simulink model "exercise_07_simscape"  (R2022b)
settings: Solver=VariableStepAuto  StartTime=0.0  StopTime=10*2*pi/w  MaxStep=(2*pi/w)*1e-4  MinStep=(2*pi/w)*1e-12  RelTol=1e-3  AbsTol=1e-3
model workspace (MAT data in the model file):
  R = 1
  X1 = 1
  X2 = 2
  XC = -1
  XM = 1
  gamma1 = 1
  gamma2 = 1
  w = 6.28318530718
libraries: fl_lib x13, nesl_utility x5
settings Model: Creator=stefa  LastModifiedBy=stefa
settings SolverCC: AutoScaleAbsTol=off  AlgebraicLoopSolver=TrustRegion  MaxZcPerStep=1
settings OptimizationCC: ReuseModelBlockBuffer=on
settings DebuggingCC: UnconnectedInputMsg=warning  UnconnectedOutputMsg=warning  UnconnectedLineMsg=warning  SymbolicDimsDataTypeCodeGenerationDiagnostic=none
settings ModelReferenceCC: EnableRefExpFcnMdlSchedulingChecks=on
settings SFSimCC: CustomCodeUndefinedFunction=UseInterfaceOnly
settings RTWCC: DLArmComputeVersion=19.05
settings SimscapeCC: SimscapeLogType=all  SimscapeLogSimulationStatistics=on  SimscapeLogDataHistory=10000

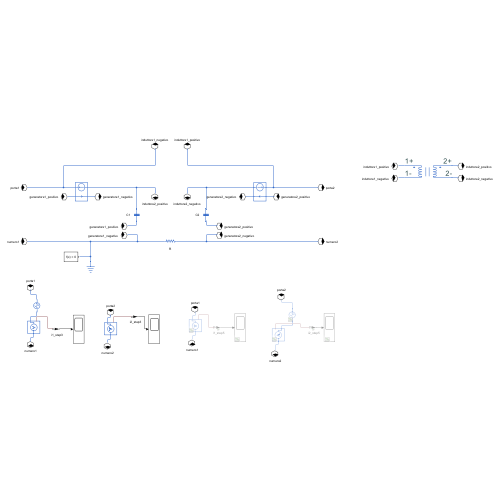
[thumbnail: Simulink's stored preview of the top-level diagram]
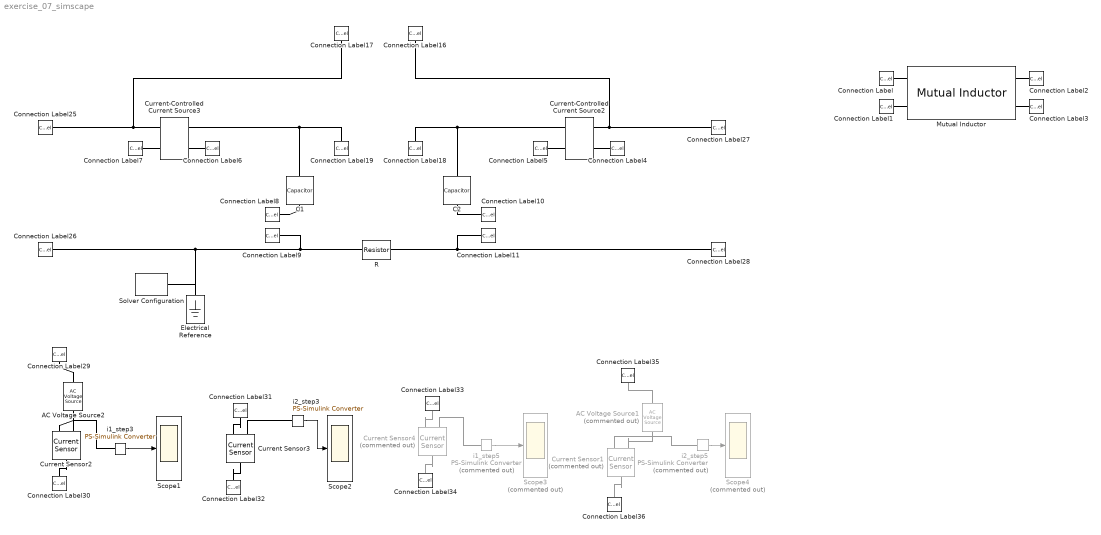
== system exercise_07_simscape ==
  AC Voltage Source1 : fl_lib/Electrical/Electrical Sources/AC Voltage Source  Commented=on  amp=1 V  shift=90 deg  frequency=w/(2*pi) Hz  omega=0 rad/s
  AC Voltage Source2 : fl_lib/Electrical/Electrical Sources/AC Voltage Source  amp=1 V  shift=90 deg  frequency=w/(2*pi) Hz  omega=0 rad/s
  C1 : fl_lib/Electrical/Electrical Elements/Capacitor  c=-1/w*XC F  r=0 Ohm  g=0 1/Ohm  i_specify=off  i_priority=None  i=0 A  i_nominal_specify=off  i_nominal_unit=A  i_nominal_value=1  v_specify=off  v_priority=None  v=0 V  v_nominal_specify=off  v_nominal_unit=V  v_nominal_value=1  vc_specify=off  vc_priority=High  vc=0 V  vc_nominal_specify=off  vc_nominal_unit=V  vc_nominal_value=1
  C2 : fl_lib/Electrical/Electrical Elements/Capacitor  c=-1/w*XC F  r=0 Ohm  g=0 1/Ohm  i_specify=off  i_priority=None  i=0 A  i_nominal_specify=off  i_nominal_unit=A  i_nominal_value=1  v_specify=off  v_priority=None  v=0 V  v_nominal_specify=off  v_nominal_unit=V  v_nominal_value=1  vc_specify=off  vc_priority=High  vc=0 V  vc_nominal_specify=off  vc_nominal_unit=V  vc_nominal_value=1
  Connection Label : ConnectionLabel  Label=induttore1_positivo
  Connection Label1 : ConnectionLabel  Label=induttore1_negativo
  Connection Label10 : ConnectionLabel  Label=generatore2_positivo
  Connection Label11 : ConnectionLabel  Label=generatore2_negativo
  Connection Label16 : ConnectionLabel  Label=induttore1_positivo
  Connection Label17 : ConnectionLabel  Label=induttore1_negativo
  Connection Label18 : ConnectionLabel  Label=induttore2_negativo
  Connection Label19 : ConnectionLabel  Label=induttore2_positivo
  Connection Label2 : ConnectionLabel  Label=induttore2_positivo
  Connection Label25 : ConnectionLabel  Label=porta1
  Connection Label26 : ConnectionLabel  Label=numero1
  Connection Label27 : ConnectionLabel  Label=porta2
  Connection Label28 : ConnectionLabel  Label=numero2
  Connection Label29 : ConnectionLabel  Label=porta1
  Connection Label3 : ConnectionLabel  Label=induttore2_negativo
  Connection Label30 : ConnectionLabel  Label=numero1
  Connection Label31 : ConnectionLabel  Label=porta2
  Connection Label32 : ConnectionLabel  Label=numero2
  Connection Label33 : ConnectionLabel  Label=porta1
  Connection Label34 : ConnectionLabel  Label=numero1
  Connection Label35 : ConnectionLabel  Label=porta2
  Connection Label36 : ConnectionLabel  Label=numero2
  Connection Label4 : ConnectionLabel  Label=generatore2_positivo
  Connection Label5 : ConnectionLabel  Label=generatore2_negativo
  Connection Label6 : ConnectionLabel  Label=generatore1_negativo
  Connection Label7 : ConnectionLabel  Label=generatore1_positivo
  Connection Label8 : ConnectionLabel  Label=generatore1_positivo
  Connection Label9 : ConnectionLabel  Label=generatore1_negativo
  Current Sensor1 : fl_lib/Electrical/Electrical Sensors/Current Sensor  Commented=on
  Current Sensor2 : fl_lib/Electrical/Electrical Sensors/Current Sensor
  Current Sensor3 : fl_lib/Electrical/Electrical Sensors/Current Sensor
  Current Sensor4 : fl_lib/Electrical/Electrical Sensors/Current Sensor  Commented=on
  Current-Controlled Current Source2 : fl_lib/Electrical/Electrical Sources/Current-Controlled Current Source  K=gamma2  i1_specify=off  i1_priority=None  i1=0 A  i1_nominal_specify=off  i1_nominal_unit=A  i1_nominal_value=1  i2_specify=off  i2_priority=None  i2=0 A  i2_nominal_specify=off  i2_nominal_unit=A  i2_nominal_value=1
      settings: InternalSimscapePortConfiguration="{\"Bottom\":[],\"Left\":[{\"id\":\"p1\",\"label\":\"+\",\"type\":\"foundation.electrical.electrical\"},{\"id\":\"head\",\"label\":\"\",\"type\":\"foundation.electrical.electrical\"}],\"Right\":[{\"id\":\"n1\",\"label\":\"-\",\"type\":\"foundation.electrical.electrical\"},{\"id\":\"tail\",\"label\":\"\",\"type\":\"foundation.electrical.electrical\"}],\"Top\":[]}"
  Current-Controlled Current Source3 : fl_lib/Electrical/Electrical Sources/Current-Controlled Current Source  K=gamma1  i1_specify=off  i1_priority=None  i1=0 A  i1_nominal_specify=off  i1_nominal_unit=A  i1_nominal_value=1  i2_specify=off  i2_priority=None  i2=0 A  i2_nominal_specify=off  i2_nominal_unit=A  i2_nominal_value=1
      settings: InternalSimscapePortConfiguration="{\"Bottom\":[],\"Left\":[{\"id\":\"p1\",\"label\":\"+\",\"type\":\"foundation.electrical.electrical\"},{\"id\":\"head\",\"label\":\"\",\"type\":\"foundation.electrical.electrical\"}],\"Right\":[{\"id\":\"n1\",\"label\":\"-\",\"type\":\"foundation.electrical.electrical\"},{\"id\":\"tail\",\"label\":\"\",\"type\":\"foundation.electrical.electrical\"}],\"Top\":[]}"
  Electrical Reference : fl_lib/Electrical/Electrical Elements/Electrical Reference
  Mutual Inductor : fl_lib/Electrical/Electrical Elements/Mutual Inductor  L1=X1/w H  L2=X2/w H  k=XM/sqrt(X1*X2)  i1_specify=off  i1_priority=High  i1=0 A  i1_nominal_specify=off  i1_nominal_unit=A  i1_nominal_value=1  i2_specify=off  i2_priority=High  i2=0 A  i2_nominal_specify=off  i2_nominal_unit=A  i2_nominal_value=1  v1_specify=off  v1_priority=None  v1=0 V  v1_nominal_specify=off  v1_nominal_unit=V  v1_nominal_value=1  v2_specify=off  v2_priority=None  v2=0 V  v2_nominal_specify=off  v2_nominal_unit=V  v2_nominal_value=1
      settings: InternalSimscapePortConfiguration="{\"Bottom\":[],\"Left\":[{\"id\":\"p1\",\"label\":\"1+\",\"type\":\"foundation.electrical.electrical\"},{\"id\":\"n1\",\"label\":\"1-\",\"type\":\"foundation.electrical.electrical\"}],\"Right\":[{\"id\":\"p2\",\"label\":\"2+\",\"type\":\"foundation.electrical.electrical\"},{\"id\":\"n2\",\"label\":\"2-\",\"type\":\"foundation.electrical.electrical\"}],\"Top\":[]}"
  R : fl_lib/Electrical/Electrical Elements/Resistor  R=R Ohm  i_specify=off  i_priority=None  i=0 A  i_nominal_specify=off  i_nominal_unit=A  i_nominal_value=1  v_specify=off  v_priority=None  v=0 V  v_nominal_specify=off  v_nominal_unit=V  v_nominal_value=1
  Scope1 : Scope
  Scope2 : Scope
  Scope3 : Scope  Commented=on
  Scope4 : Scope  Commented=on
  Solver Configuration : nesl_utility/Solver Configuration  PhysicalDomain=network_engine_domain  SubClassName=solver  LeftPortType=input  RightPortType=generic  Tones=[]  Harmonics=[]  SimulateNoise=off  Profile=off  UseLocalSampling=off  EnableSwitchedLinearOptims=on  FrequencyDomain=off  UseCCode=off  RelTol=0.001  AbsTol=0.001  MinStep=1e-09  ToWorkspace=off  RevertToSquareIcSolve=off  NumHomotopyIterations=100  PhasorMode=off  PhasorModeNumHarmonics=1  ConsistencySolver=NEWTON_XTOL_AFTER_FTOL  IndexReductionMethod=DerivativeReplacement  DoDC=off  ResidualTolerance=1e-09  ConsistencyTolSource=GLOBAL  ConsistencyAbsTol=0.001  ConsistencyRelTol=0.001  ConsistencyTolFactor=0.001  UseLocalSolver=off  LocalSolverChoice=NE_BACKWARD_EULER_ADVANCER  ResolveIndetEquations=on  FunctionEvalNumThread=1  LocalSolverSampleTime=0.001  DoFixedCost=off  MaxNonlinIter=3  MaxModeIter=2  ComputeImpulses=off  ImpulseIterations=2  LinearAlgebra=auto  LinearAlgebraNumThread=0  EquationFormulation=NE_TIME_EF  DelaysMemoryBudget=1024  AutomaticFiltering=on  FilteringTimeConstant=0.001  PartitionStorageMethod=AS_NEEDED  PartitionMemoryBudget=1024  PartitionMethod=ROBUST
  i1_step3 : nesl_utility/PS-Simulink Converter  PhysicalDomain=network_engine_domain  SubClassName=ps_output  LeftPortType=input  RightPortType=output  PseudoPeriodic=off  Frequencies=[]  VectorFormat=1-D array  Unit=inherit  AffineConversion=off
  i1_step5 : nesl_utility/PS-Simulink Converter  Commented=on  PhysicalDomain=network_engine_domain  SubClassName=ps_output  LeftPortType=input  RightPortType=output  PseudoPeriodic=off  Frequencies=[]  VectorFormat=1-D array  Unit=inherit  AffineConversion=off
  i2_step3 : nesl_utility/PS-Simulink Converter  PhysicalDomain=network_engine_domain  SubClassName=ps_output  LeftPortType=input  RightPortType=output  PseudoPeriodic=off  Frequencies=[]  VectorFormat=1-D array  Unit=inherit  AffineConversion=off
  i2_step5 : nesl_utility/PS-Simulink Converter  Commented=on  PhysicalDomain=network_engine_domain  SubClassName=ps_output  LeftPortType=input  RightPortType=output  PseudoPeriodic=off  Frequencies=[]  VectorFormat=1-D array  Unit=inherit  AffineConversion=off
  wires:
  i1_step5/1 -> Scope3/1
  i2_step3/1 -> Scope2/1
  i1_step3/1 -> Scope1/1
  i2_step5/1 -> Scope4/1
  connections:
  Current Sensor4/LConn1 -- Connection Label34/LConn1
  Connection Label32/LConn1 -- Current Sensor3/LConn1
  Current Sensor2/RConn1 -- i1_step3/LConn1
  Current Sensor3/RConn1 -- i2_step3/LConn1
  Current Sensor1/RConn1 -- i2_step5/LConn1
  Current Sensor2/LConn1 -- Connection Label30/LConn1
  AC Voltage Source2/RConn1 -- Current Sensor2/RConn2
  Current Sensor4/RConn1 -- i1_step5/LConn1
  Current Sensor1/LConn1 -- Connection Label36/LConn1
  Current Sensor4/RConn2 -- Connection Label33/LConn1
  AC Voltage Source1/LConn1 -- Connection Label35/LConn1
  Connection Label31/LConn1 -- Current Sensor3/RConn2
  AC Voltage Source2/LConn1 -- Connection Label29/LConn1
  Current Sensor1/RConn2 -- AC Voltage Source1/RConn1
  Connection Label/LConn1 -- Mutual Inductor/LConn1
  Connection Label1/LConn1 -- Mutual Inductor/LConn2
  Connection Label2/LConn1 -- Mutual Inductor/RConn1
  Connection Label3/LConn1 -- Mutual Inductor/RConn2
  Current-Controlled Current Source3/RConn1 -- Connection Label6/LConn1
  Connection Label7/LConn1 -- Current-Controlled Current Source3/LConn1
  Current-Controlled Current Source3/RConn2 -- Connection Label19/LConn1 -- C1/LConn1
  Current-Controlled Current Source3/LConn2 -- Connection Label17/LConn1 -- Connection Label25/LConn1
  Connection Label5/LConn1 -- Current-Controlled Current Source2/RConn1
  Connection Label4/LConn1 -- Current-Controlled Current Source2/LConn1
  C2/LConn1 -- Connection Label18/LConn1 -- Current-Controlled Current Source2/RConn2
  Current-Controlled Current Source2/LConn2 -- Connection Label27/LConn1 -- Connection Label16/LConn1
  R/LConn1 -- Connection Label9/LConn1 -- Solver Configuration/RConn1 -- Electrical Reference/LConn1 -- Connection Label26/LConn1
  R/RConn1 -- Connection Label11/LConn1 -- Connection Label28/LConn1
  Connection Label8/LConn1 -- C1/RConn1
  C2/RConn1 -- Connection Label10/LConn1
